simulink model "oneDim"  (R2022b)
settings: Solver=FixedStepAuto  StartTime=0.0  StopTime=30  FixedStep=dt  RelTol=1e-3
values from neighbouring files (symbols this model uses):
  Cd = 0.5    [oneDim_mfile.m]
  D_adm = 2*zeta_adm*wn_adm*M_adm    (= 20)    [DC_motor_mfile.m]    (also in oneDim_mfile.m = 1)
  D_imp = 2*zeta_imp*wn_imp*m    (= 50)    [oneDim_mfile.m]
  g = 9.807    [DC_motor_mfile.m]    (also in oneDim_mfile.m)
  K_adm = wn_adm^2*M_adm    (= 100)    [DC_motor_mfile.m]    (also in oneDim_mfile.m = 2.5)
  K_imp = wn_imp^2 * m    (= 1250)    [oneDim_mfile.m]
  m = 1    [DC_motor_mfile.m]    (also in oneDim_mfile.m = 0.5)
  M_adm = 1    [DC_motor_mfile.m]    (also in oneDim_mfile.m = 0.1)
  rho_air = 1.225    [oneDim_mfile.m]
  S = pi*0.2^2    (= 0.125663706144)    [oneDim_mfile.m]
settings Model: Creator=chris  LastModifiedBy=chris

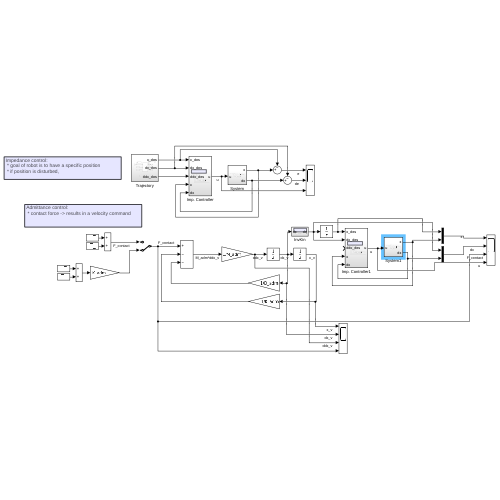
[thumbnail: Simulink's stored preview of the top-level diagram]
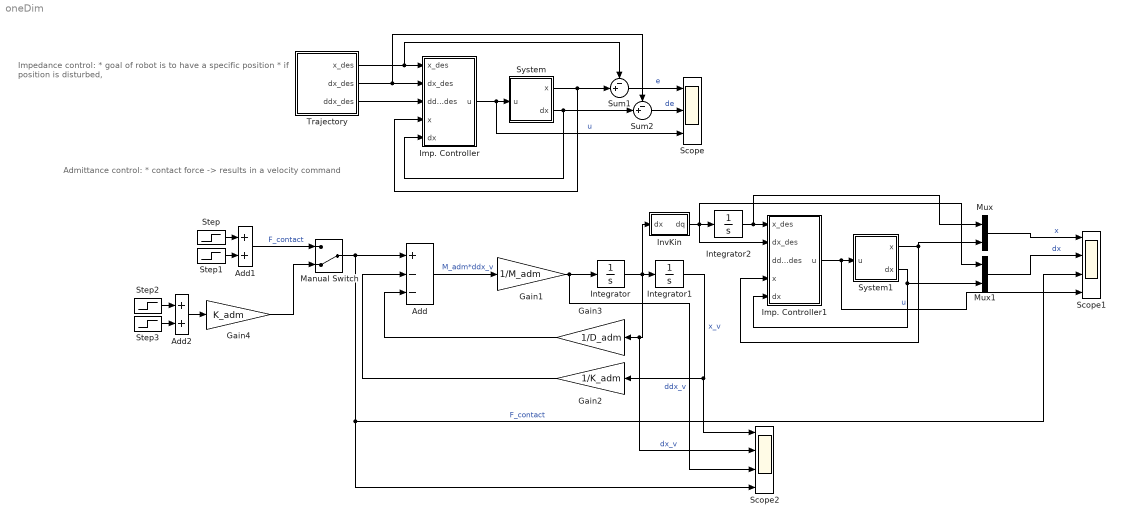
== system oneDim ==
  note: Impedance control:
      |  * goal of robot is to have a specific position
      |  * if position is disturbed,
  note: Admittance control:
      |  * contact force -> results in a velocity command
  Add : Sum  Inputs=+--
  Add1 : Sum
  Add2 : Sum
  Gain1 : Gain  Gain=1/M_adm
  Gain2 : Gain  Gain=1/K_adm
  Gain3 : Gain  Gain=1/D_adm
  Gain4 : Gain  Gain=K_adm
  Imp. Controller : Subsystem
  Imp. Controller1 : Subsystem
  Integrator : Integrator
  Integrator1 : Integrator
  Integrator2 : Integrator
  InvKin : Subsystem
  Manual Switch : ManualSwitch  CurrentSetting=0
  Mux : Mux  Inputs=2
  Mux1 : Mux  Inputs=2
  Scope : Scope  NumInputPorts=3
  Scope1 : Scope  NumInputPorts=4
  Scope2 : Scope  NumInputPorts=4
  Step : Step  Time=5  SampleTime=0
  Step1 : Step  Time=15  After=-1  SampleTime=0
  Step2 : Step  Time=5  SampleTime=0
  Step3 : Step  Time=15  After=-1  SampleTime=0
  Sum1 : Sum  Inputs=-+|
  Sum2 : Sum  Inputs=-+|
  System : Subsystem
  System1 : Subsystem
  Trajectory : Subsystem
  wires:
  System/1(x) -> Sum1/2, Imp. Controller/4(x)
  System/2(dx) -> Sum2/2, Imp. Controller/5(dx)
  Imp. Controller/1(u) -> Scope/3, System/1(u)  "u"
  Trajectory/1(x_des) -> Sum1/1, Imp. Controller/1(x_des)
  Trajectory/2(dx_des) -> Sum2/1, Imp. Controller/2(dx_des)
  Trajectory/3(ddx_des) -> Imp. Controller/3(ddx_des)
  Sum1/1 -> Scope/1  "e"
  Sum2/1 -> Scope/2  "de"
  Add/1 -> Gain1/1  "M_adm*ddx_v"
  Gain1/1 -> Scope2/3, Integrator/1  "ddx_v"
  Integrator1/1 -> Scope2/1, Gain2/1  "x_v"
  Integrator/1 -> InvKin/1(dx), Scope2/2, Gain3/1, Integrator1/1  "dx_v"
  Gain2/1 -> Add/2
  Gain3/1 -> Add/3
  Manual Switch/1 -> Add/1, Scope1/3, Scope2/4  "F_contact"
  Integrator2/1 -> Mux/1, Imp. Controller1/1(x_des)
  Imp. Controller1/1(u) -> Scope1/4, System1/1(u)  "u"
  System1/1(x) -> Mux/2, Imp. Controller1/4(x)
  System1/2(dx) -> Mux1/2, Imp. Controller1/5(dx)
  Mux/1 -> Scope1/1  "x"
  Mux1/1 -> Scope1/2  "dx"
  InvKin/1(dq) -> Imp. Controller1/2(dx_des), Mux1/1, Integrator2/1
  Step/1 -> Add1/1
  Step1/1 -> Add1/2
  Add1/1 -> Manual Switch/1  "F_contact"
  Gain4/1 -> Manual Switch/2
  Add2/1 -> Gain4/1
  Step2/1 -> Add2/1
  Step3/1 -> Add2/2

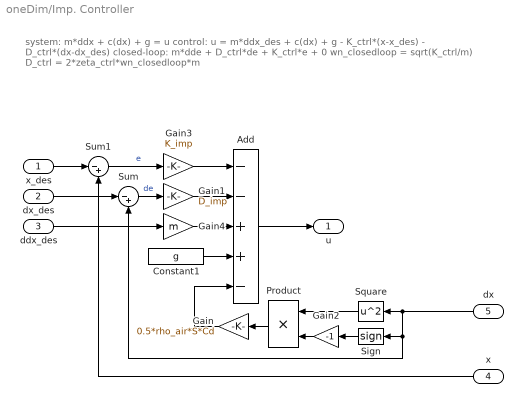
== system oneDim/Imp. Controller ==
  note: system: m*ddx + c(dx) + g = u
      | control: u = m*ddx_des + c(dx) + g - K_ctrl*(x-x_des) - D_ctrl*(dx-dx_des)
      | closed-loop: m*dde + D_ctrl*de + K_ctrl*e + 0
      |
      | wn_closedloop = sqrt(K_ctrl/m)
      | D_ctrl = 2*zeta_ctrl*wn_closedloop*m
  x_des : Inport
  dx_des : Inport  Port=2
  ddx_des : Inport  Port=3
  x : Inport  Port=4
  dx : Inport  Port=5
  Add : Sum  Inputs=--++-
  Constant1 : Constant  Value=g
  Gain : Gain  Gain=0.5*rho_air*S*Cd
  Gain1 : Gain  Gain=D_imp
  Gain2 : Gain  Gain=-1
  Gain3 : Gain  Gain=K_imp
  Gain4 : Gain  Gain=m
  Product : Product
  Sign : Signum
  Square : Math  Operator=square
  Sum : Sum  Inputs=|-+
  Sum1 : Sum  Inputs=|-+
  u : Outport
  wires:
  Constant1/1 -> Add/4
  x/1 -> Sum1/2
  Gain2/1 -> Product/2
  ddx_des/1 -> Gain4/1
  Sum/1 -> Gain1/1  "de"
  Sign/1 -> Gain2/1
  Gain/1 -> Add/5
  x_des/1 -> Sum1/1
  dx_des/1 -> Sum/1
  Sum1/1 -> Gain3/1  "e"
  Gain4/1 -> Add/3
  Gain1/1 -> Add/2
  Gain3/1 -> Add/1
  Add/1 -> u/1
  Square/1 -> Product/1
  Product/1 -> Gain/1
  dx/1 -> Square/1, Sign/1, Sum/2

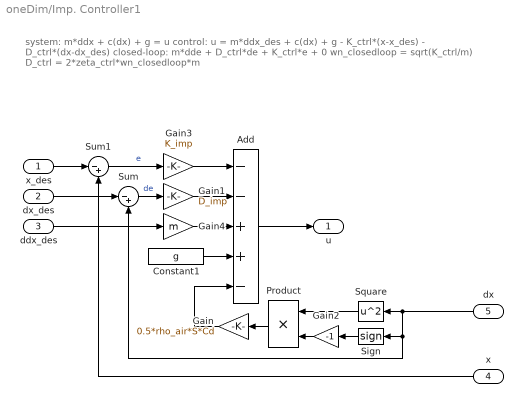
== system oneDim/Imp. Controller1 ==
  note: system: m*ddx + c(dx) + g = u
      | control: u = m*ddx_des + c(dx) + g - K_ctrl*(x-x_des) - D_ctrl*(dx-dx_des)
      | closed-loop: m*dde + D_ctrl*de + K_ctrl*e + 0
      |
      | wn_closedloop = sqrt(K_ctrl/m)
      | D_ctrl = 2*zeta_ctrl*wn_closedloop*m
  x_des : Inport
  dx_des : Inport  Port=2
  ddx_des : Inport  Port=3
  x : Inport  Port=4
  dx : Inport  Port=5
  Add : Sum  Inputs=--++-
  Constant1 : Constant  Value=g
  Gain : Gain  Gain=0.5*rho_air*S*Cd
  Gain1 : Gain  Gain=D_imp
  Gain2 : Gain  Gain=-1
  Gain3 : Gain  Gain=K_imp
  Gain4 : Gain  Gain=m
  Product : Product
  Sign : Signum
  Square : Math  Operator=square
  Sum : Sum  Inputs=|-+
  Sum1 : Sum  Inputs=|-+
  u : Outport
  wires:
  Constant1/1 -> Add/4
  x/1 -> Sum1/2
  Gain2/1 -> Product/2
  ddx_des/1 -> Gain4/1
  Sum/1 -> Gain1/1  "de"
  Sign/1 -> Gain2/1
  Gain/1 -> Add/5
  x_des/1 -> Sum1/1
  dx_des/1 -> Sum/1
  Sum1/1 -> Gain3/1  "e"
  Gain4/1 -> Add/3
  Gain1/1 -> Add/2
  Gain3/1 -> Add/1
  Add/1 -> u/1
  Square/1 -> Product/1
  Product/1 -> Gain/1
  dx/1 -> Square/1, Sign/1, Sum/2

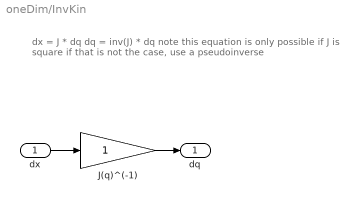
== system oneDim/InvKin ==
  note: dx = J * dq
      | dq = inv(J) * dq
      |
      | note this equation is only possible if J is square
      | if that is not the case, use a pseudoinverse
  dx : Inport
  J(q)^(-1) : Gain
  dq : Outport
  wires:
  J(q)^(-1)/1 -> dq/1
  dx/1 -> J(q)^(-1)/1

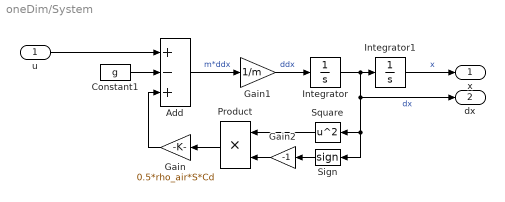
== system oneDim/System ==
  u : Inport
  Add : Sum  Inputs=+-+
  Constant1 : Constant  Value=g
  Gain : Gain  Gain=0.5*rho_air*S*Cd
  Gain1 : Gain  Gain=1/m
  Gain2 : Gain  Gain=-1
  Integrator : Integrator
  Integrator1 : Integrator
  Product : Product
  Sign : Signum
  Square : Math  Operator=square
  x : Outport
  dx : Outport  Port=2
  wires:
  Constant1/1 -> Add/2
  Gain/1 -> Add/3
  Add/1 -> Gain1/1  "m*ddx"
  Sign/1 -> Gain2/1
  Gain1/1 -> Integrator/1  "ddx"
  Gain2/1 -> Product/2
  Square/1 -> Product/1
  Product/1 -> Gain/1
  u/1 -> Add/1
  Integrator/1 -> dx/1, Sign/1, Square/1, Integrator1/1  "dx"
  Integrator1/1 -> x/1  "x"

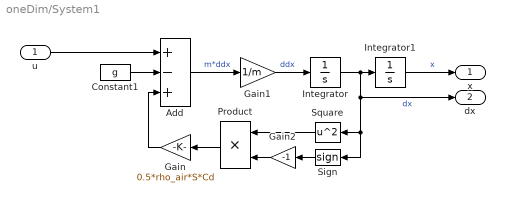
== system oneDim/System1 ==
  u : Inport
  Add : Sum  Inputs=+-+
  Constant1 : Constant  Value=g
  Gain : Gain  Gain=0.5*rho_air*S*Cd
  Gain1 : Gain  Gain=1/m
  Gain2 : Gain  Gain=-1
  Integrator : Integrator
  Integrator1 : Integrator
  Product : Product
  Sign : Signum
  Square : Math  Operator=square
  x : Outport
  dx : Outport  Port=2
  wires:
  Constant1/1 -> Add/2
  Gain/1 -> Add/3
  Add/1 -> Gain1/1  "m*ddx"
  Sign/1 -> Gain2/1
  Gain1/1 -> Integrator/1  "ddx"
  Gain2/1 -> Product/2
  Square/1 -> Product/1
  Product/1 -> Gain/1
  u/1 -> Add/1
  Integrator/1 -> dx/1, Sign/1, Square/1, Integrator1/1  "dx"
  Integrator1/1 -> x/1  "x"

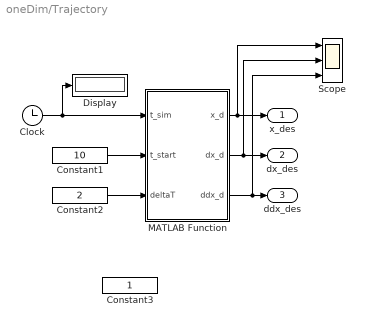
== system oneDim/Trajectory ==
  Clock : Clock
  Constant1 : Constant  Value=10
  Constant2 : Constant  Value=2
  Constant3 : Constant
  Display : Display
  MATLAB Function : MATLAB Function  TreatAsAtomicUnit=on
  Scope : Scope  NumInputPorts=3
  x_des : Outport
  dx_des : Outport  Port=2
  ddx_des : Outport  Port=3
  wires:
  MATLAB Function/3(ddx_d) -> Scope/3, ddx_des/1
  MATLAB Function/1(x_d) -> Scope/1, x_des/1
  MATLAB Function/2(dx_d) -> Scope/2, dx_des/1
  Clock/1 -> Display/1, MATLAB Function/1(t_sim)
  Constant1/1 -> MATLAB Function/2(t_start)
  Constant2/1 -> MATLAB Function/3(deltaT)

== matlab function oneDim/Trajectory/MATLAB Function ==
  data: t_sim input; x_d output; dx_d output; ddx_d output; t_start input; deltaT input
function [x_d,dx_d,ddx_d] = fcn(t_sim,t_start,deltaT)

t = t_sim - t_start;
acc = 2*9.807;
if (t>=0 && t<=deltaT)
    x_d = 0.5*acc*(t-0)^2 + 0*(t-0) + 0;
    dx_d = acc*(t-0) + 0;
    ddx_d = acc;
elseif (t>deltaT && t<=2*deltaT)
    s_temp = 0.5*acc*deltaT^2;
    V_temp = acc*deltaT;
    x_d = V_temp*(t-deltaT) + s_temp;
    dx_d = V_temp;
    ddx_d = 0;
elseif (t>2*deltaT && t<=4*deltaT)
    s_temp = 0.5*acc*deltaT^2 + (acc*deltaT)*deltaT;
    V_temp = acc*deltaT;
    x_d = -0.5*acc*(t-2*deltaT)^2 + V_temp*(t-2*deltaT) + s_temp;
    dx_d = V_temp - acc*(t-2*deltaT);
    ddx_d = -acc;
elseif (t>4*deltaT && t<=5*deltaT)
    s_temp = 0.5*acc*deltaT^2 + (acc*deltaT)*deltaT;
    V_temp = -acc*deltaT;
    x_d = s_temp+V_temp*(t-4*deltaT);
    dx_d = V_temp;
    ddx_d = 0;
elseif (t>5*deltaT && t<=6*deltaT)
    s_temp = 0.5*acc*deltaT^2;
    V_temp = -acc*deltaT;
    x_d = 0.5*acc*(t-5*deltaT)^2 + V_temp*(t-5*deltaT) + s_temp;
    dx_d = acc*(t-5*deltaT) + V_temp;
    ddx_d = acc;
else
    x_d = 0;
    dx_d = 0;
    ddx_d = 0;
end
